simulink subsystem "WindGFMTurbineInertia23a"  (R2023a)
settings: Solver=VariableStepAuto  StartTime=0.0  StopTime=10.0  RelTol=1e-3
model mask{Kp=0, D=0, H=0, KqI=0, Vd_ref=0, frequency=0, x_vir=0, r_vir=0, Imax=0, Radius1=0, pitch1=0, cp1=0, TSR1=0, airDensity1=0, wt1=0, rt1=0, Inertia1=0, p1=0, psim1=0, Ld1=0, Lq1=0, Rs1=0, Kp_dc_sm=0, Ki_dc_sm=0, Kpd=0, Kid=0, Kpq=0, Kiq=0}
  mask prompts: Kp "VSM frequency droop"; D "VSM damping"; H "VSM Inertia"; KqI "VSM Reactive power droop"; Vd_ref "Volatge Reference d-axis"; frequency "Reference frequency"; x_vir "Virtual reactance"; r_vir "Virtual resistance"; Imax "Current limit"; Radius1 "Radius of Turbine"; pitch1 "Pitch Angle Vector"; cp1 "Power Coefficient Table"; TSR1 "Tip Speed Ratio"; airDensity1 "Air Density"; wt1 "Wind Velocity Threshold"; rt1 "Rotational Velocity Threshold"; Inertia1 "Turbine Inertia"; p1 "Number of Pole Pairs"; psim1 "PM Flux Linkage"; Ld1 "Stator D-axis inductance (H)"; Lq1 "Stator Q-axis inductance (H)"; Rs1 "Stator Resistance (Ohms)"; Kp_dc_sm "Prportional Gain of Dc-link Controller"; Ki_dc_sm "Integral Gain of DC-link Controller"; Kpd "D-axis proportional Gain"; Kid "D-axis integral Gain"; Kpq "q-axis proportional Gain"; Kiq "q-axis integral Gain"
undefined symbols (not defined in the file): alpha, base, DiscIntNeverNeededParam, Ld, Lq, mpptPower, mpptWindSpeed, p, psim, Rs, Ts, windController, windInverter, windTurbine
libraries: nesl_utility x14, ee_lib x9, fl_lib x7, slpidlib x5, eeTransforms x5, eeGeneralControl x2, simulink x2, eePowerMeasurement x1, eePmsmCurrentController x1
(part 2 of 2)

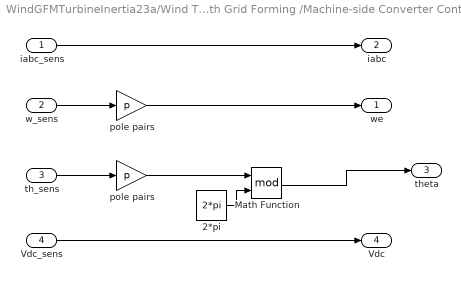
== system WindGFMTurbineInertia23a/Wind Turbine with Grid Forming /Machine-side Converter Control/Measurements ==
  iabc_sens : Inport
  w_sens : Inport  Port=2
  th_sens : Inport  Port=3
  Vdc_sens : Inport  Port=4
  2*pi : Constant  Value=2*pi  SampleTime=-1
  Math Function : Math  Operator=mod  SignedPower=on
  pole pairs : Gain  Gain=p
  "pole pairs " : Gain  Gain=p
  we : Outport  VectorParamsAs1DForOutWhenUnconnected=off
  iabc : Outport  Port=2  VectorParamsAs1DForOutWhenUnconnected=off
  theta : Outport  Port=3  VectorParamsAs1DForOutWhenUnconnected=off
  Vdc : Outport  Port=4  VectorParamsAs1DForOutWhenUnconnected=off
  wires:
  w_sens/1 -> pole pairs/1
  iabc_sens/1 -> iabc/1
  pole pairs/1 -> we/1
  2*pi/1 -> Math Function/2
  th_sens/1 -> "pole pairs "/1
  "pole pairs "/1 -> Math Function/1
  Vdc_sens/1 -> Vdc/1
  Math Function/1 -> theta/1

== system WindGFMTurbineInertia23a/Wind Turbine with Grid Forming /PMSG/Meas I ==
  Current Sensor : ee_lib/Sensors & Transducers/Current Sensor (Three-Phase)
  PS-Simulink Converter : nesl_utility/PS-Simulink Converter  PhysicalDomain=network_engine_domain  SubClassName=ps_output  LeftPortType=input  RightPortType=output  PseudoPeriodic=off  Frequencies=[]  VectorFormat=inherit  Unit=A  AffineConversion=off
  1 : PMIOPort  Side=Left
  2 : PMIOPort  Port=2  Side=Right
  iabc : Outport
  wires:
  PS-Simulink Converter/1 -> iabc/1
  connections:
  Current Sensor/RConn1 -- PS-Simulink Converter/LConn1
  Current Sensor/LConn1 -- 1/RConn1
  Current Sensor/RConn2 -- 2/RConn1

== system WindGFMTurbineInertia23a/Wind Turbine with Grid Forming /Power Controller/Derating Control ==
  Enable : EnablePort  StatesWhenEnabling=reset
  Constant : Constant  Value=windTurbine.turbineRatedPower
  MW to W : Gain  Gain=1e6
  activePowerDemand : Outport
  wires:
  MW to W/1 -> activePowerDemand/1
  Constant/1 -> MW to W/1

== system WindGFMTurbineInertia23a/Wind Turbine with Grid Forming /Power Controller/Limiter Function Power Demand ==
  activePowerDemandMPPT : Inport
  activePowerDemandDerating : Inport  Port=2
  Merge : Merge
  activePowerDemand : Outport
  wires:
  activePowerDemandMPPT/1 -> Merge/1
  activePowerDemandDerating/1 -> Merge/2
  Merge/1 -> activePowerDemand/1

== system WindGFMTurbineInertia23a/Wind Turbine with Grid Forming /Power Controller/MPPT Control ==
  windSpeed : Inport
  Enable : EnablePort  StatesWhenEnabling=reset
  MW to W : Gain  Gain=1e6
  mpptActivePowerDemand : Lookup_n-D  NumberOfTableDimensions=1  BreakpointsForDimension1=mpptWindSpeed  Table=mpptPower*4  InternalRulePriority=Speed  RndMeth=Simplest
  activePowerDemand : Outport
  wires:
  mpptActivePowerDemand/1 -> MW to W/1
  windSpeed/1 -> mpptActivePowerDemand/1
  MW to W/1 -> activePowerDemand/1
